simulink model "o03M_POROWNANIE_CIAGLY_DYSKRETNY_EULER"  (R2023a)
settings: Solver=ode45  StartTime=0.0  StopTime=5  RelTol=1e-3
values from neighbouring files (symbols this model uses):
  calka_on_off = 1    [o03S_skrypt_prownanie.m]
  den_f_e = sym2poly(d)    [o03S_skrypt_prownanie.m]
  fsz = 2500    [o03S_skrypt_prownanie.m]
  Jeq = JL + J    (= 3.228252e-05)    [o03S_skrypt_prownanie.m]
  K_windup = 3    [o03S_skrypt_prownanie.m]
  Km = 0.0257    [o03S_skrypt_prownanie.m]
  Kp = 0.04    [o03S_skrypt_prownanie.m]
  num_f_e = sym2poly(n)    [o03S_skrypt_prownanie.m]
  Psz = 0.005    [o03S_skrypt_prownanie.m]
  Rm = 2.675    [o03S_skrypt_prownanie.m]
  Td = 0.009    [o03S_skrypt_prownanie.m]
  Ti = 0.11    [o03S_skrypt_prownanie.m]
  Ts = 1/fs    (= 0.0333333333333)    [o03S_skrypt_prownanie.m]
  w_filtr = 10    [o03S_skrypt_prownanie.m]
undefined symbols (not defined in the file or in its folder): sigbuilder_block
libraries: simulink x2
settings Model: Creator=Adam  LastModifiedBy=Adam
settings SolverCC: ZeroCrossAlgorithm=Adaptive  AlgebraicLoopSolver=TrustRegion
settings DebuggingCC: IgnoredZcDiagnostic=none  UnconnectedInputMsg=warning  UnconnectedOutputMsg=warning  UnconnectedLineMsg=warning
settings ModelReferenceCC: EnableRefExpFcnMdlSchedulingChecks=on
settings RTWCC: DLArmComputeVersion=19.05

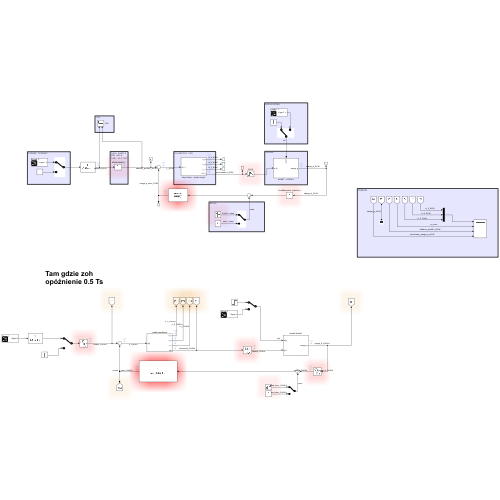
[thumbnail: Simulink's stored preview of the top-level diagram]
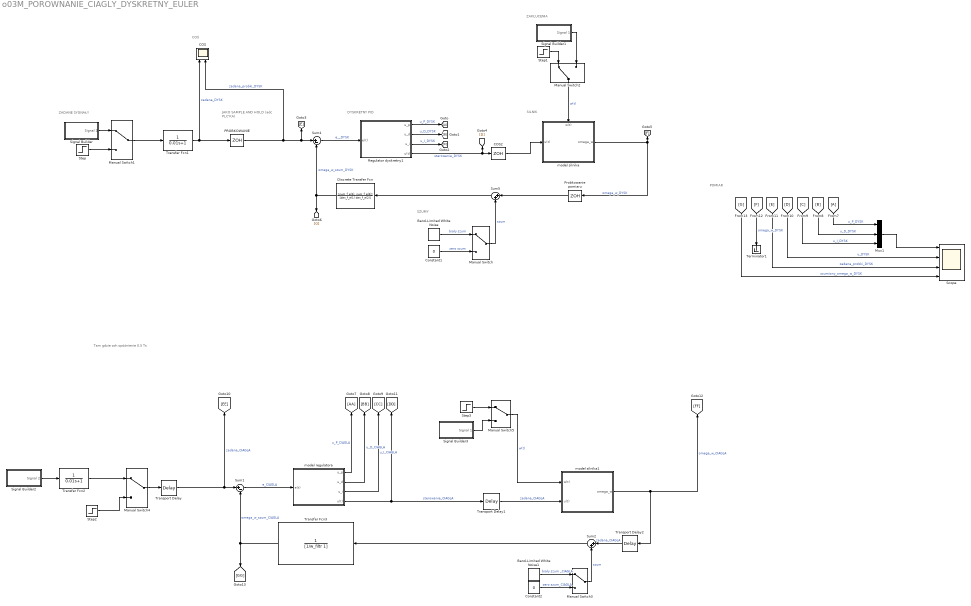
== system o03M_POROWNANIE_CIAGLY_DYSKRETNY_EULER ==
  note: Tam gdzie zoh opóźnienie 0.5 Ts
  note: ZAKŁUCENIA
  note: POMIAR
  note: SZUMY
  note: JAKO SAMPLE
      | AND HOLD
      | (adc PLC'KA)
  note: SILNIK
  note: DYSKRETNY PID
  note: COŚ
  note: ZADANE SYGNAŁY
  Band-Limited White Noise : simulink/Sources/Band-Limited White Noise  Cov=[Psz]  Ts=0.1  seed=[fsz]
  Band-Limited White Noise1 : simulink/Sources/Band-Limited White Noise  Cov=[Psz]  Ts=0.1  seed=[fsz]
  "COS " : Scope  NumInputPorts=2
  COS2 : ZeroOrderHold  SampleTime=Ts
  Constant1 : Constant  Value=0
  Constant2 : Constant  Value=0
  Discrete Transfer Fcn : DiscreteTransferFcn  Numerator=[num_f_e(1), num_f_e(2)]  Denominator=[den_f_e(1) den_f_e(2)]  SampleTime=Ts
  From7 : From
  Goto : Goto
  Manual Switch{,1..5} (6 alike) : ManualSwitch
  Mux1 : Mux  Inputs=3
  PROBKOWANIE : ZeroOrderHold  SampleTime=Ts
  Probkowanie pomiaru : ZeroOrderHold  SampleTime=Ts
  Regulator dyskretny1 : Subsystem
  Scope : Scope  NumInputPorts=4
  Signal Builder : Subsystem  Tag=STV Subsys  LoadFcn=sigbuilder_block('load');  StartFcn=sigbuilder_block('start');  StopFcn=sigbuilder_block('stop');  ClipboardFcn=sigbuilder_block('clipboard');  mask(Sigbuilder block){tuvar=[0:10]}
      mask help: Simulink:masks:SigbuilderBlock_MD
      mask init:
      | if ~strcmp(get_param(bdroot(gcbh),'SimulationStatus'),'stopped') tuvar = sigbuilder_block('maskInit'); end
      settings: CopyFcn=sigbuilder_block('copy');  DeleteFcn=sigbuilder_block('delete');  ModelCloseFcn=sigbuilder_block('modelClose');  PreSaveFcn=sigbuilder_block('preSave');  PauseFcn=sigbuilder_block('pause');  ContinueFcn=sigbuilder_block('continue');  NameChangeFcn=sigbuilder_block('namechange');  OpenFcn=sigbuilder_block('open',[261 231 1018.5 399.75 ]);  CloseFcn=sigbuilder_block('close');
      mask Display: plot(0, 0, 100, 100,[2, 2, 32, 32, 2], [68, 8, 8, 68, 68],[32, 2], [38, 38], [32, 19, 2],[53, 60, 44], [32, 17, 17, 2],[16, 16, 31, 31]);txt = getActiveGroup(gcbh);text(2, 100, txt,'verticalAlignment', 'top');
  Signal Builder1 : Subsystem  Tag=STV Subsys  LoadFcn=sigbuilder_block('load');  StartFcn=sigbuilder_block('start');  StopFcn=sigbuilder_block('stop');  ClipboardFcn=sigbuilder_block('clipboard');  mask(Sigbuilder block){tuvar=[0:10]}
      mask help: Simulink:masks:SigbuilderBlock_MD
      mask init:
      | if ~strcmp(get_param(bdroot(gcbh),'SimulationStatus'),'stopped') tuvar = sigbuilder_block('maskInit'); end
      settings: CopyFcn=sigbuilder_block('copy');  DeleteFcn=sigbuilder_block('delete');  ModelCloseFcn=sigbuilder_block('modelClose');  PreSaveFcn=sigbuilder_block('preSave');  PauseFcn=sigbuilder_block('pause');  ContinueFcn=sigbuilder_block('continue');  NameChangeFcn=sigbuilder_block('namechange');  OpenFcn=sigbuilder_block('open',[261 231 1018.5 399.75 ]);  CloseFcn=sigbuilder_block('close');
      mask Display: plot(0, 0, 100, 100,[2, 2, 32, 32, 2], [68, 8, 8, 68, 68],[32, 2], [38, 38], [32, 19, 2],[53, 60, 44], [32, 17, 17, 2],[16, 16, 31, 31]);txt = getActiveGroup(gcbh);text(2, 100, txt,'verticalAlignment', 'top');
  Signal Builder2 : Subsystem  Tag=STV Subsys  LoadFcn=sigbuilder_block('load');  StartFcn=sigbuilder_block('start');  StopFcn=sigbuilder_block('stop');  ClipboardFcn=sigbuilder_block('clipboard');  mask(Sigbuilder block){tuvar=[0:10]}
      mask help: Simulink:masks:SigbuilderBlock_MD
      mask init:
      | if ~strcmp(get_param(bdroot(gcbh),'SimulationStatus'),'stopped') tuvar = sigbuilder_block('maskInit'); end
      settings: CopyFcn=sigbuilder_block('copy');  DeleteFcn=sigbuilder_block('delete');  ModelCloseFcn=sigbuilder_block('modelClose');  PreSaveFcn=sigbuilder_block('preSave');  PauseFcn=sigbuilder_block('pause');  ContinueFcn=sigbuilder_block('continue');  NameChangeFcn=sigbuilder_block('namechange');  OpenFcn=sigbuilder_block('open',[261 231 1018.5 399.75 ]);  CloseFcn=sigbuilder_block('close');
      mask Display: plot(0, 0, 100, 100,[2, 2, 32, 32, 2], [68, 8, 8, 68, 68],[32, 2], [38, 38], [32, 19, 2],[53, 60, 44], [32, 17, 17, 2],[16, 16, 31, 31]);txt = getActiveGroup(gcbh);text(2, 100, txt,'verticalAlignment', 'top');
  Signal Builder3 : Subsystem  Tag=STV Subsys  LoadFcn=sigbuilder_block('load');  StartFcn=sigbuilder_block('start');  StopFcn=sigbuilder_block('stop');  ClipboardFcn=sigbuilder_block('clipboard');  mask(Sigbuilder block){tuvar=[0:10]}
      mask help: Simulink:masks:SigbuilderBlock_MD
      mask init:
      | if ~strcmp(get_param(bdroot(gcbh),'SimulationStatus'),'stopped') tuvar = sigbuilder_block('maskInit'); end
      settings: CopyFcn=sigbuilder_block('copy');  DeleteFcn=sigbuilder_block('delete');  ModelCloseFcn=sigbuilder_block('modelClose');  PreSaveFcn=sigbuilder_block('preSave');  PauseFcn=sigbuilder_block('pause');  ContinueFcn=sigbuilder_block('continue');  NameChangeFcn=sigbuilder_block('namechange');  OpenFcn=sigbuilder_block('open',[261 231 1018.5 399.75 ]);  CloseFcn=sigbuilder_block('close');
      mask Display: plot(0, 0, 100, 100,[2, 2, 32, 32, 2], [68, 8, 8, 68, 68],[32, 2], [38, 38], [32, 19, 2],[53, 60, 44], [32, 17, 17, 2],[16, 16, 31, 31]);txt = getActiveGroup(gcbh);text(2, 100, txt,'verticalAlignment', 'top');
  Step : Step  SampleTime=0
  Step1 : Step  Time=2  After=0.03  SampleTime=0
  Step2 : Step  SampleTime=0
  Step3 : Step  Time=2  After=0.03  SampleTime=0
  Sum1 : Sum  Inputs=|+-
  Sum2 : Sum  Inputs=|++
  Sum4 : Sum  Inputs=|+-
  Sum5 : Sum  Inputs=|++
  Terminator1 : Terminator
  Transfer Fcn1 : TransferFcn  Denominator=[0.01 1]
  Transfer Fcn2 : TransferFcn  Denominator=[0.01 1]
  Transfer Fcn3 : TransferFcn  Denominator=[1/w_filtr 1]
  Transport Delay : TransportDelay  DelayTime=Ts/2
  Transport Delay1 : TransportDelay  DelayTime=Ts/2
  Transport Delay2 : TransportDelay  DelayTime=Ts/2
  model regulatora : Subsystem
  model silnika : Subsystem
      settings: PortSchema="{\"entries\":[{\"content\":{\"sides\":[{\"content\":{\"connectorIds\":[\"In1\"]},\"type\":\"ConnectorPlacement.EquallySpacedRectSide\",\"uuid\":\"98491aef-0591-4405-8c9c-40e364f6fd31\"},{\"content\":{\"connectorIds\":[\"Out1\"],\"side\":\"RIGHT\"},\"type\":\"ConnectorPlacement.EquallySpacedRectSide\",\"uuid\":\"a1d3aa00-38e6-4d5e-ba9e-ca8054307f42\"},{\"content\":{\"connectorIds\":[\"In2\"],\"side\":\"TOP\"},\"type\":\"ConnectorPlacement.EquallySpacedRectSide\",\"uuid\":\"056a3762-abf1-4492-b9c7-e5ea07edcbab\"},{\"content\":{\"connectorIds\":[],\"side\":\"HIDDEN\"},\"type\":\"ConnectorPlacement.EquallySpacedRectSide\",\"uuid\":\"0c2ff021-be20-4132-8d80-585248c3a111\"}]},\"type\":\"ConnectorPlacement.EquallySpacedConnector\",\"uuid\":\"f7102573-6331-4f02-a900-8db50f80a4fd\"}],\"packageUris\":[\"http://schema.mathworks.com/mf0/Connector/R2020b\"],\"version\":\"1.0\"}"
  model silnika1 : Subsystem
  wires:
  Band-Limited White Noise/1 -> Manual Switch/1  "biały szum"
  Constant1/1 -> Manual Switch/2  "zero szum"
  model silnika/1(omega_w) -> Probkowanie pomiaru/1, [F]  "omega_w_DYSK"
  Manual Switch/1 -> Sum5/2  "szum"
  Signal Builder/1(Signal 2) -> Manual Switch1/1
  Step/1 -> Manual Switch1/2
  [G] -> Scope/4  "szumiony_omega_w_DYSK"
  [C] -> Mux1/3  "u_I_DYSK"
  [E] -> Scope/3  "zadana_probki_DYSK"
  [D] -> Scope/2  "u_DYSK"
  From7/1 -> Mux1/1  "u_P_DYSK"
  [B] -> Mux1/2  "u_D_DYSK"
  Mux1/1 -> Scope/1
  [F] -> Terminator1/1  "omega_w_DYSK"
  Regulator dyskretny1/3(u_i) -> [C]  "u_I_DYSK"
  Regulator dyskretny1/1(u_p) -> Goto/1  "u_P_DYSK"
  Regulator dyskretny1/4(u(t)) -> [D], COS2/1  "sterowanie_DYSK"
  Sum4/1 -> Regulator dyskretny1/1(e(t))  "e__DYSK"
  Regulator dyskretny1/2(u_d) -> [B]  "u_D_DYSK"
  Sum5/1 -> Discrete Transfer Fcn/1
  Step1/1 -> Manual Switch2/1
  Signal Builder1/1(Signal 1) -> Manual Switch2/2
  PROBKOWANIE/1 -> "COS "/2, Sum4/1, [E]  "zadana_probki_DYSK"
  Probkowanie pomiaru/1 -> Sum5/1
  COS2/1 -> model silnika/1(u(t))
  Transfer Fcn1/1 -> PROBKOWANIE/1, "COS "/1  "zadana_DYSK"
  Manual Switch1/1 -> Transfer Fcn1/1
  Manual Switch2/1 -> model silnika/2(w(t))  "w(t)"
  Discrete Transfer Fcn/1 -> [G], Sum4/2  "omega_w_szum_DYSK"
  Sum1/1 -> model regulatora/1(e(t))  "e_CIAGLA"
  model silnika1/1(omega_w) -> Transport Delay2/1, [FF]  "omega_w_CIAGLA"
  Manual Switch5/1 -> model silnika1/1(w(t))  "w(t)"
  Constant2/1 -> Manual Switch3/2  "zero szum_CIAGLA"
  Signal Builder3/1(Signal 1) -> Manual Switch5/2
  model regulatora/1(u_p) -> [AA]  "u_P_CIAGLA"
  Step2/1 -> Manual Switch4/2
  Signal Builder2/1(Signal 2) -> Transfer Fcn2/1
  Manual Switch3/1 -> Sum2/2  "szum"
  Transfer Fcn2/1 -> Manual Switch4/1
  model regulatora/2(u_d) -> [BB]  "u_D_CIAGLA"
  Step3/1 -> Manual Switch5/1
  Transfer Fcn3/1 -> [GG], Sum1/2  "omega_w_szum_CIAGLA"
  model regulatora/3(u_i) -> [CC]  "u_I_CIAGLA"
  model regulatora/4(u(t)) -> [DD], Transport Delay1/1  "sterowanie_CIAGLA"
  Manual Switch4/1 -> Transport Delay/1
  Sum2/1 -> Transfer Fcn3/1
  Band-Limited White Noise1/1 -> Manual Switch3/1  "biały szum _CIAGLA"
  Transport Delay/1 -> [EE], Sum1/1  "zadana_CIAGLA"
  Transport Delay1/1 -> model silnika1/2(u(t))  "zadana_CIAGLA"
  Transport Delay2/1 -> Sum2/1  "zadana_CIAGLA"

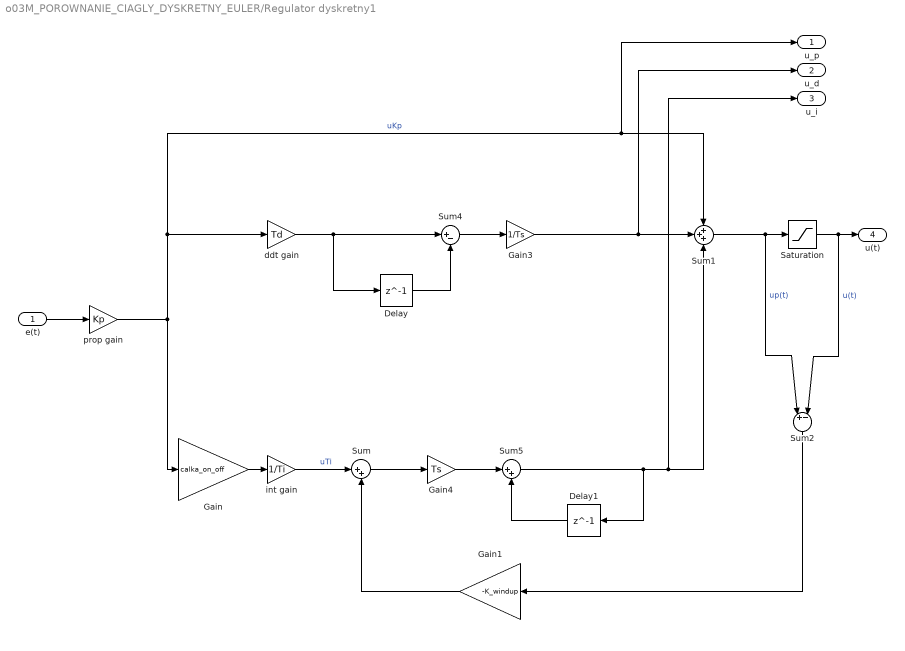
== system o03M_POROWNANIE_CIAGLY_DYSKRETNY_EULER/Regulator dyskretny1 ==
  e(t) : Inport
  Delay : Delay  DelayLength=1  SampleTime=Ts
  Delay1 : Delay  DelayLength=1  SampleTime=Ts
  Gain : Gain  Gain=calka_on_off
  Gain1 : Gain  Gain=-K_windup
  Gain3 : Gain  Gain=1/Ts
  Gain4 : Gain  Gain=Ts
  Saturation : Saturate  UpperLimit=10  LowerLimit=-10  ZeroCross=off
  Sum : Sum  Inputs=|++
  Sum1 : Sum  Inputs=+++
  Sum2 : Sum  Inputs=|+-|
  Sum4 : Sum  Inputs=|+-
  Sum5 : Sum  Inputs=|++
  ddt gain : Gain  Gain=Td
  int gain : Gain  Gain=1/Ti
  prop gain : Gain  Gain=Kp
  u_p : Outport
  u_d : Outport  Port=2
  u_i : Outport  Port=3
  u(t) : Outport  Port=4
  wires:
  Sum1/1 -> Sum2/1, Saturation/1  "up(t)"
  prop gain/1 -> Sum1/1, u_p/1, ddt gain/1, Gain/1  "uKp"
  Saturation/1 -> Sum2/2, u(t)/1  "u(t)"
  e(t)/1 -> prop gain/1
  Gain/1 -> int gain/1
  int gain/1 -> Sum/1  "uTi"
  Gain1/1 -> Sum/2
  Sum2/1 -> Gain1/1
  ddt gain/1 -> Delay/1, Sum4/1
  Delay/1 -> Sum4/2
  Sum4/1 -> Gain3/1
  Sum/1 -> Gain4/1
  Gain3/1 -> u_d/1, Sum1/2
  Gain4/1 -> Sum5/1
  Delay1/1 -> Sum5/2
  Sum5/1 -> Delay1/1, u_i/1, Sum1/3

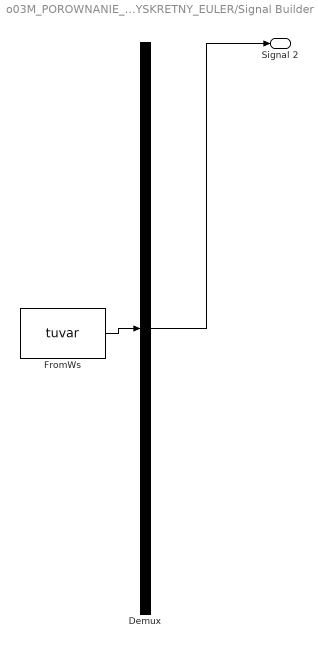
== system o03M_POROWNANIE_CIAGLY_DYSKRETNY_EULER/Signal Builder ==
  Demux : Demux  Tag=STV Demux  Outputs=1
      settings: DisplayOption=none
  FromWs : FromWorkspace  Tag=STV FromWs  VariableName=tuvar
      SigBuilderData=|
      | common.afterFinalStr = 'Extrapolate'
      | common.sampleTime = 0
      | dataSet.timeRange = [0 25]
      | dataSet.name = 'Group 1'
      | sbobj.Groups.Name = 'Group 1'
      | sbobj.Groups.Signals.Name = 'Signal 2'
      | sbobj.Groups.Signals.XData = [0 4 4 9.2 9.2 14 14 25]
      | sbobj.Groups.Signals.YData = [100 100 -150 -150 -100 -100 150 150]
      | sbobj.Groups.TimeRange = [0 25]
  Signal 2 : Outport  Tag=STV Outport
  wires:
  FromWs/1 -> Demux/1
  Demux/1 -> Signal 2/1

== system o03M_POROWNANIE_CIAGLY_DYSKRETNY_EULER/Signal Builder1 ==
  Demux : Demux  Tag=STV Demux  Outputs=1
      settings: DisplayOption=none
  FromWs : FromWorkspace  Tag=STV FromWs  VariableName=tuvar
      SigBuilderData=|
      | common.afterFinalStr = 'Extrapolate'
      | common.sampleTime = 0
      | dataSet.timeRange = [0 25]
      | dataSet.name = 'Group 1'
      | sbobj.Groups.Name = 'Group 1'
      | sbobj.Groups.Signals.Name = 'Signal 1'
      | sbobj.Groups.Signals.XData = [0 2.05 2.05 4.05 4.05 6 6 8 8 16 16 18 18 25]
      | sbobj.Groups.Signals.YData = [0 0 0.075 0.075 -0.001 -0.001 -0.0775 -0.0775 0 0 0.075 0.075 0 0]
      | sbobj.Groups.TimeRange = [0 25]
  Signal 1 : Outport  Tag=STV Outport
  wires:
  FromWs/1 -> Demux/1
  Demux/1 -> Signal 1/1

== system o03M_POROWNANIE_CIAGLY_DYSKRETNY_EULER/Signal Builder2 ==
  Demux : Demux  Tag=STV Demux  Outputs=1
      settings: DisplayOption=none
  FromWs : FromWorkspace  Tag=STV FromWs  VariableName=tuvar
      SigBuilderData=|
      | common.afterFinalStr = 'Extrapolate'
      | common.sampleTime = 0
      | dataSet.timeRange = [0 25]
      | dataSet.name = 'Group 1'
      | sbobj.Groups.Name = 'Group 1'
      | sbobj.Groups.Signals.Name = 'Signal 2'
      | sbobj.Groups.Signals.XData = [0 4 4 9.2 9.2 14 14 25]
      | sbobj.Groups.Signals.YData = [100 100 -150 -150 -100 -100 150 150]
      | sbobj.Groups.TimeRange = [0 25]
  Signal 2 : Outport  Tag=STV Outport
  wires:
  FromWs/1 -> Demux/1
  Demux/1 -> Signal 2/1

== system o03M_POROWNANIE_CIAGLY_DYSKRETNY_EULER/Signal Builder3 ==
  Demux : Demux  Tag=STV Demux  Outputs=1
      settings: DisplayOption=none
  FromWs : FromWorkspace  Tag=STV FromWs  VariableName=tuvar
      SigBuilderData=|
      | common.afterFinalStr = 'Extrapolate'
      | common.sampleTime = 0
      | dataSet.timeRange = [0 25]
      | dataSet.name = 'Group 1'
      | sbobj.Groups.Name = 'Group 1'
      | sbobj.Groups.Signals.Name = 'Signal 1'
      | sbobj.Groups.Signals.XData = [0 2.05 2.05 4.05 4.05 6 6 8 8 16 16 18 18 25]
      | sbobj.Groups.Signals.YData = [0 0 0.075 0.075 -0.001 -0.001 -0.0775 -0.0775 0 0 0.075 0.075 0 0]
      | sbobj.Groups.TimeRange = [0 25]
  Signal 1 : Outport  Tag=STV Outport
  wires:
  FromWs/1 -> Demux/1
  Demux/1 -> Signal 1/1

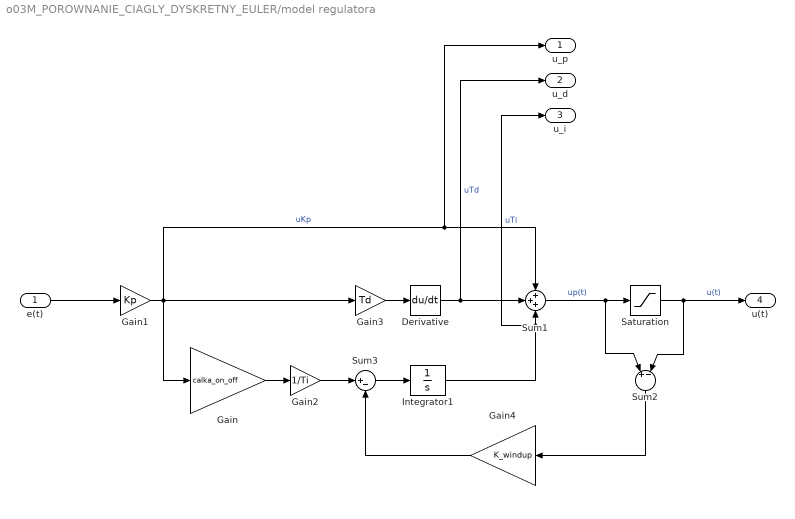
== system o03M_POROWNANIE_CIAGLY_DYSKRETNY_EULER/model regulatora ==
  e(t) : Inport
  Derivative : Derivative  CoefficientInTFapproximation=500
  Gain : Gain  Gain=calka_on_off
  Gain1 : Gain  Gain=Kp
  Gain2 : Gain  Gain=1/Ti
  Gain3 : Gain  Gain=Td
  Gain4 : Gain  Gain=K_windup
  Integrator1 : Integrator
  Saturation : Saturate  UpperLimit=10  LowerLimit=-10  ZeroCross=off
  Sum1 : Sum  Inputs=+++
  Sum2 : Sum  Inputs=|+-|
  Sum3 : Sum  Inputs=|+-
  u_p : Outport
  u_d : Outport  Port=2
  u_i : Outport  Port=3
  u(t) : Outport  Port=4
  wires:
  Sum1/1 -> Sum2/1, Saturation/1  "up(t)"
  Gain2/1 -> Sum3/1
  Sum2/1 -> Gain4/1
  Derivative/1 -> u_d/1, Sum1/2  "uTd"
  Gain3/1 -> Derivative/1
  Gain1/1 -> Gain/1, Gain3/1, u_p/1, Sum1/1  "uKp"
  Integrator1/1 -> u_i/1, Sum1/3  "uTi"
  Sum3/1 -> Integrator1/1
  Saturation/1 -> u(t)/1, Sum2/2  "u(t)"
  e(t)/1 -> Gain1/1
  Gain/1 -> Gain2/1
  Gain4/1 -> Sum3/2

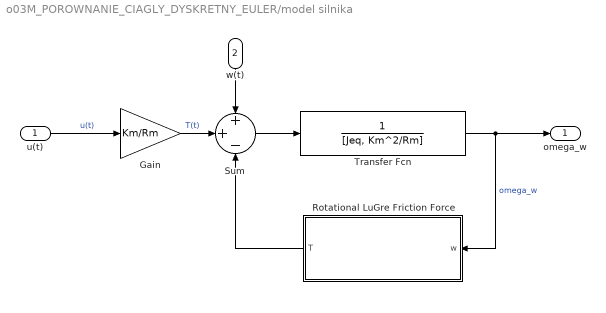
== system o03M_POROWNANIE_CIAGLY_DYSKRETNY_EULER/model silnika ==
  u(t) : Inport
  w(t) : Inport  Port=2
  Gain : Gain  Gain=Km/Rm
  Rotational LuGre Friction Force : Subsystem  TreatAsAtomicUnit=on  mask(LuGre friction model){ro0=1.2, ro1=0.05, ro2=2.9e-6, Fc=0.77e-3, Fs=12e-3, Vs=0.09}
      mask prompts: Fc "Culomb force (Fc)"; Fs "Friction force (Fs)"; Vs "Striback velocity (Vs)"
      mask help:
      | The LuGre model is a dynamic friction model. The model is related to the bristle interpretation of friction. Friction is modeled as the average deflection force of elastic springs. When a tangential force is applied the bristles will deflect like springs. If the deflection is sufficiently large the bristles start to slip.
      |
      | The input signal is the velocity of the object. The output signal is the fristion force value.
      mask Help:
      | <!DOCTYPE html   PUBLIC "-//W3C//DTD HTML 4.01 Transitional//EN" "http://www.w3.org/TR/1999/REC-html401-19991224/loose.dtd">
      | <html lang="en"><head>
      | <meta http-equiv="Content-Type" content="text/html; charset=utf-8">
      | <title>About :: LuGre friction model</title>
      | <meta name="description" content="">
      | </head>
      | <body><a name="top_of_page"></a>
      | The LuGre model is a dynamic friction model. The model is related to
      | the bristle interpretation of friction. Friction is modeled as the average
      | deflection force of elastic springs. When a tangential force is applied the bristles
      | will deflect like springs. If the deflection is sufficiently large the bristles start
      | to slip. The average bristle deflection for a steady state motion is determined
      | by the velocity. It is lower at low velocities, which implies that the steady state
      | deflection decreases with increasing velocity. This models the phenomenon that
      | the surfaces are pushed apart by the lubricant, and models the Stribeck effect.
      | The model also includes rate dependent friction phenomena such as varying
      | break-away force and frictional lag.<sup><a href="#ref1">1</a></sup></p><p>More information about the model may be found in the labsheets.</p>
      | <hr><small>
      | <sup><a name="ref1"></a>1</sup> <b>Friction Models and Friction Compensation</b>. H. Olsson, K.J. &Aring;str&ouml;m, C. Canudas de Wit, M. G&auml;fvert, P. Lischinsky
      | </small>
      | <br />
      | <br />
      | <hr>
      | <center><small>Copyright&copy;2009
      | <a href="mailto:w.kurek@ely.pg.gda.pl">Wojciech Kurek</a>,
      | <a href="mailto:g.ewald@ely.pg.gda.pl">Grzegorz Ewald</a>
      | </small></center>
      | </body>
      | </html>
      mask Callback ro0:
      | if str2num(get_param(gcb, 'ro0')) <= 0
      |     error('ro0 is negative!')
      | end
      mask Callback ro1:
      | if str2num(get_param(gcb, 'ro1')) <= 0
      |     error('ro1 is negative!')
      | end
      mask Callback ro2:
      | if str2num(get_param(gcb, 'ro2')) <= 0
      |     error('ro2 is negative!')
      | end
      mask Callback Fc:
      | if str2num(get_param(gcb, 'Fs')) <= 0
      |     error('Culomb force is negative!')
      | end
      mask Callback Fs:
      | if str2num(get_param(gcb, 'Fs')) <= 0
      |     error('Friction force is negative!')
      | end
      mask Callback Vs:
      | if str2num(get_param(gcb, 'Vs')) <= 0
      |     error('Striback velocity is negative!')
      | end
      mask Display:
      | patch([0.1 0.1 0.9 0.9],[0.1 0.25 0.25 0.1],[0.8 0.8 0.8])
      | patch([0.1 0.1 0.9 0.9],[0.9 0.75 0.75 0.9],[0.8 0.8 0.8])
      | 
      | plot([0.12 0.12],[0.25 0.5])
      | plot([0.2 0.2],[0.25 0.5])
      | plot([0.4 0.4],[0.25 0.5])
      | plot([0.57 0.57],[0.25 0.5])
      | plot([0.67 0.67],[0.25 0.5])
      | plot([0.87 0.87],[0.25 0.5])
      | 
      | plot([0.17 0.18 0.2 0.23],[0.75 0.6 0.5 0.45])
      | plot([0.35 0.36 0.39 0.44],[0.75 0.6 0.5 0.48])
      | plot([0.62 0.64 0.68 0.72],[0.75 0.6 0.5 0.48])
      | plot([0.85 0.86 0.87 0.89],[0.75 0.6 0.5 0.48])
      | 
      | plot([0.15 0.15],[0.75 0.4])
      | plot([0.28 0.28],[0.75 0.4])
      | plot([0.55 0.55],[0.75 0.4])
      | plot([0.8 0.8],[0.75 0.4])
      | 
      | color('blue');
      | port_label('input',1,'\omega','texmode','on')
      | port_label('output',1,'T','texmode','on')
  Sum : Sum  Inputs=++-
  Transfer Fcn : TransferFcn  Denominator=[Jeq, Km^2/Rm]
  omega_w : Outport
  wires:
  Transfer Fcn/1 -> Rotational LuGre Friction Force/1(w), omega_w/1  "omega_w"
  Rotational LuGre Friction Force/1(T) -> Sum/3
  Sum/1 -> Transfer Fcn/1
  Gain/1 -> Sum/2  "T(t)"
  u(t)/1 -> Gain/1  "u(t)"
  w(t)/1 -> Sum/1

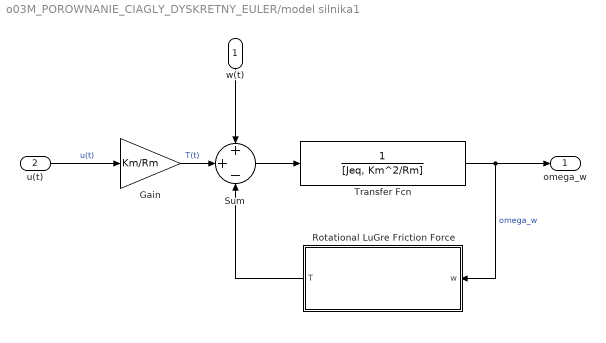
== system o03M_POROWNANIE_CIAGLY_DYSKRETNY_EULER/model silnika1 ==
  w(t) : Inport
  u(t) : Inport  Port=2
  Gain : Gain  Gain=Km/Rm
  Rotational LuGre Friction Force : Subsystem  TreatAsAtomicUnit=on  mask(LuGre friction model){ro0=1.2, ro1=0.05, ro2=2.9e-6, Fc=0.77e-3, Fs=12e-3, Vs=0.09}
      mask prompts: Fc "Culomb force (Fc)"; Fs "Friction force (Fs)"; Vs "Striback velocity (Vs)"
      mask help:
      | The LuGre model is a dynamic friction model. The model is related to the bristle interpretation of friction. Friction is modeled as the average deflection force of elastic springs. When a tangential force is applied the bristles will deflect like springs. If the deflection is sufficiently large the bristles start to slip.
      |
      | The input signal is the velocity of the object. The output signal is the fristion force value.
      mask Help:
      | <!DOCTYPE html   PUBLIC "-//W3C//DTD HTML 4.01 Transitional//EN" "http://www.w3.org/TR/1999/REC-html401-19991224/loose.dtd">
      | <html lang="en"><head>
      | <meta http-equiv="Content-Type" content="text/html; charset=utf-8">
      | <title>About :: LuGre friction model</title>
      | <meta name="description" content="">
      | </head>
      | <body><a name="top_of_page"></a>
      | The LuGre model is a dynamic friction model. The model is related to
      | the bristle interpretation of friction. Friction is modeled as the average
      | deflection force of elastic springs. When a tangential force is applied the bristles
      | will deflect like springs. If the deflection is sufficiently large the bristles start
      | to slip. The average bristle deflection for a steady state motion is determined
      | by the velocity. It is lower at low velocities, which implies that the steady state
      | deflection decreases with increasing velocity. This models the phenomenon that
      | the surfaces are pushed apart by the lubricant, and models the Stribeck effect.
      | The model also includes rate dependent friction phenomena such as varying
      | break-away force and frictional lag.<sup><a href="#ref1">1</a></sup></p><p>More information about the model may be found in the labsheets.</p>
      | <hr><small>
      | <sup><a name="ref1"></a>1</sup> <b>Friction Models and Friction Compensation</b>. H. Olsson, K.J. &Aring;str&ouml;m, C. Canudas de Wit, M. G&auml;fvert, P. Lischinsky
      | </small>
      | <br />
      | <br />
      | <hr>
      | <center><small>Copyright&copy;2009
      | <a href="mailto:w.kurek@ely.pg.gda.pl">Wojciech Kurek</a>,
      | <a href="mailto:g.ewald@ely.pg.gda.pl">Grzegorz Ewald</a>
      | </small></center>
      | </body>
      | </html>
      mask Callback ro0:
      | if str2num(get_param(gcb, 'ro0')) <= 0
      |     error('ro0 is negative!')
      | end
      mask Callback ro1:
      | if str2num(get_param(gcb, 'ro1')) <= 0
      |     error('ro1 is negative!')
      | end
      mask Callback ro2:
      | if str2num(get_param(gcb, 'ro2')) <= 0
      |     error('ro2 is negative!')
      | end
      mask Callback Fc:
      | if str2num(get_param(gcb, 'Fs')) <= 0
      |     error('Culomb force is negative!')
      | end
      mask Callback Fs:
      | if str2num(get_param(gcb, 'Fs')) <= 0
      |     error('Friction force is negative!')
      | end
      mask Callback Vs:
      | if str2num(get_param(gcb, 'Vs')) <= 0
      |     error('Striback velocity is negative!')
      | end
      mask Display:
      | patch([0.1 0.1 0.9 0.9],[0.1 0.25 0.25 0.1],[0.8 0.8 0.8])
      | patch([0.1 0.1 0.9 0.9],[0.9 0.75 0.75 0.9],[0.8 0.8 0.8])
      | 
      | plot([0.12 0.12],[0.25 0.5])
      | plot([0.2 0.2],[0.25 0.5])
      | plot([0.4 0.4],[0.25 0.5])
      | plot([0.57 0.57],[0.25 0.5])
      | plot([0.67 0.67],[0.25 0.5])
      | plot([0.87 0.87],[0.25 0.5])
      | 
      | plot([0.17 0.18 0.2 0.23],[0.75 0.6 0.5 0.45])
      | plot([0.35 0.36 0.39 0.44],[0.75 0.6 0.5 0.48])
      | plot([0.62 0.64 0.68 0.72],[0.75 0.6 0.5 0.48])
      | plot([0.85 0.86 0.87 0.89],[0.75 0.6 0.5 0.48])
      | 
      | plot([0.15 0.15],[0.75 0.4])
      | plot([0.28 0.28],[0.75 0.4])
      | plot([0.55 0.55],[0.75 0.4])
      | plot([0.8 0.8],[0.75 0.4])
      | 
      | color('blue');
      | port_label('input',1,'\omega','texmode','on')
      | port_label('output',1,'T','texmode','on')
  Sum : Sum  Inputs=++-
  Transfer Fcn : TransferFcn  Denominator=[Jeq, Km^2/Rm]
  omega_w : Outport
  wires:
  Transfer Fcn/1 -> Rotational LuGre Friction Force/1(w), omega_w/1  "omega_w"
  Rotational LuGre Friction Force/1(T) -> Sum/3
  w(t)/1 -> Sum/1
  Sum/1 -> Transfer Fcn/1
  Gain/1 -> Sum/2  "T(t)"
  u(t)/1 -> Gain/1  "u(t)"

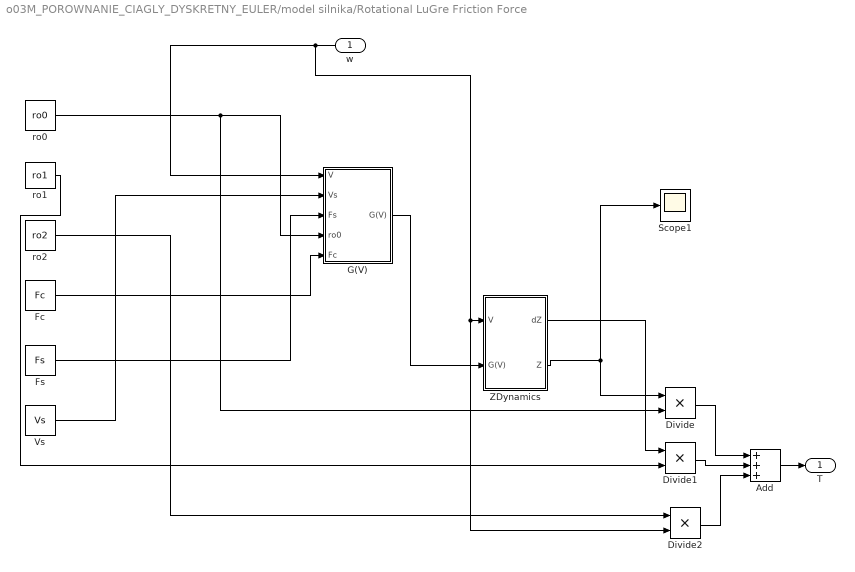
== system o03M_POROWNANIE_CIAGLY_DYSKRETNY_EULER/model silnika/Rotational LuGre Friction Force ==
  w : Inport
  Add : Sum  Inputs=+++
  Divide : Product  Inputs=**
  Divide1 : Product  Inputs=**
  Divide2 : Product  Inputs=**
  Fc : Constant  Value=Fc
  Fs : Constant  Value=Fs
  G(V) : Subsystem
  Scope1 : Scope
  Vs : Constant  Value=Vs
  ZDynamics : Subsystem
  ro0 : Constant  Value=ro0
  ro1 : Constant  Value=ro1
  ro2 : Constant  Value=ro2
  T : Outport
  wires:
  Add/1 -> T/1
  Divide2/1 -> Add/3
  Divide1/1 -> Add/2
  Divide/1 -> Add/1
  ro2/1 -> Divide2/1
  ro1/1 -> Divide1/2
  ZDynamics/1(dZ) -> Divide1/1
  ZDynamics/2(Z) -> Scope1/1, Divide/1
  G(V)/1(G(V)) -> ZDynamics/2(G(V))
  ro0/1 -> Divide/2, G(V)/4(ro0)
  Fc/1 -> G(V)/5(Fc)
  Fs/1 -> G(V)/3(Fs)
  Vs/1 -> G(V)/2(Vs)
  w/1 -> G(V)/1(V), ZDynamics/1(V), Divide2/2

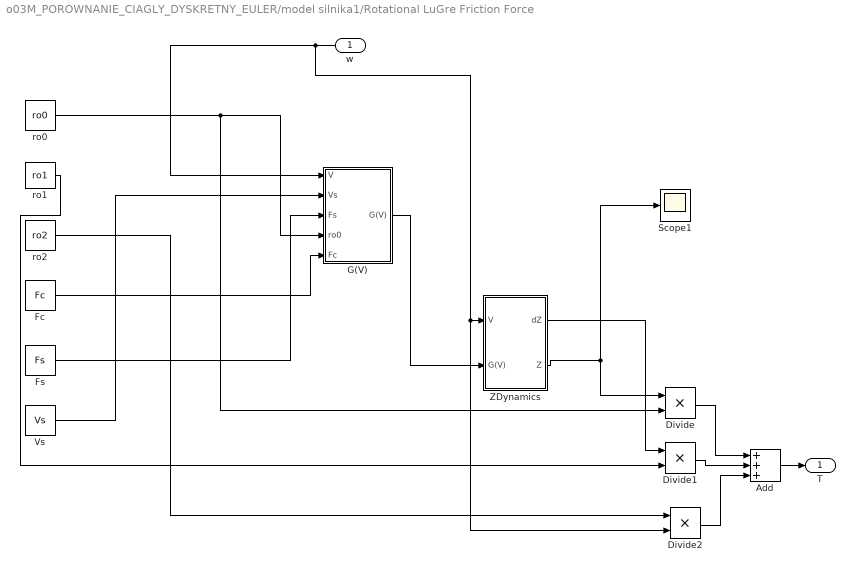
== system o03M_POROWNANIE_CIAGLY_DYSKRETNY_EULER/model silnika1/Rotational LuGre Friction Force ==
  w : Inport
  Add : Sum  Inputs=+++
  Divide : Product  Inputs=**
  Divide1 : Product  Inputs=**
  Divide2 : Product  Inputs=**
  Fc : Constant  Value=Fc
  Fs : Constant  Value=Fs
  G(V) : Subsystem
  Scope1 : Scope
  Vs : Constant  Value=Vs
  ZDynamics : Subsystem
  ro0 : Constant  Value=ro0
  ro1 : Constant  Value=ro1
  ro2 : Constant  Value=ro2
  T : Outport
  wires:
  Add/1 -> T/1
  Divide2/1 -> Add/3
  Divide1/1 -> Add/2
  Divide/1 -> Add/1
  ro2/1 -> Divide2/1
  ro1/1 -> Divide1/2
  ZDynamics/1(dZ) -> Divide1/1
  ZDynamics/2(Z) -> Scope1/1, Divide/1
  G(V)/1(G(V)) -> ZDynamics/2(G(V))
  ro0/1 -> Divide/2, G(V)/4(ro0)
  Fc/1 -> G(V)/5(Fc)
  Fs/1 -> G(V)/3(Fs)
  Vs/1 -> G(V)/2(Vs)
  w/1 -> G(V)/1(V), ZDynamics/1(V), Divide2/2

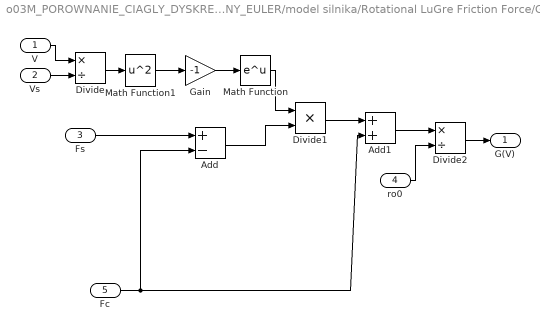
== system o03M_POROWNANIE_CIAGLY_DYSKRETNY_EULER/model silnika/Rotational LuGre Friction Force/G(V) ==
  V : Inport
  Vs : Inport  Port=2
  Fs : Inport  Port=3
  ro0 : Inport  Port=4
  Fc : Inport  Port=5
  Add : Sum  Inputs=+-
  Add1 : Sum
  Divide : Product  Inputs=*/
  Divide1 : Product  Inputs=**
  Divide2 : Product  Inputs=*/
  Gain : Gain  Gain=-1
  Math Function : Math  SignedPower=on
  Math Function1 : Math  Operator=square  SignedPower=on
  G(V) : Outport
  wires:
  Math Function/1 -> Divide1/1
  Gain/1 -> Math Function/1
  Math Function1/1 -> Gain/1
  ro0/1 -> Divide2/2
  Divide2/1 -> G(V)/1
  Fs/1 -> Add/1
  Vs/1 -> Divide/2
  V/1 -> Divide/1
  Add1/1 -> Divide2/1
  Divide1/1 -> Add1/1
  Add/1 -> Divide1/2
  Fc/1 -> Add/2, Add1/2
  Divide/1 -> Math Function1/1

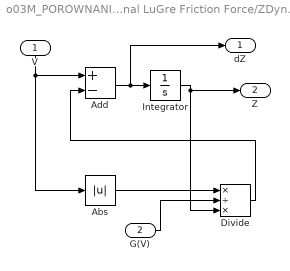
== system o03M_POROWNANIE_CIAGLY_DYSKRETNY_EULER/model silnika/Rotational LuGre Friction Force/ZDynamics ==
  V : Inport
  G(V) : Inport  Port=2
  Abs : Abs  SaturateOnIntegerOverflow=off
  Add : Sum  Inputs=+-
  Divide : Product  Inputs=*/*
  Integrator : Integrator
  dZ : Outport
  Z : Outport  Port=2
  wires:
  G(V)/1 -> Divide/2
  V/1 -> Abs/1, Add/1
  Divide/1 -> Add/2
  Integrator/1 -> Z/1, Divide/3
  Abs/1 -> Divide/1
  Add/1 -> dZ/1, Integrator/1

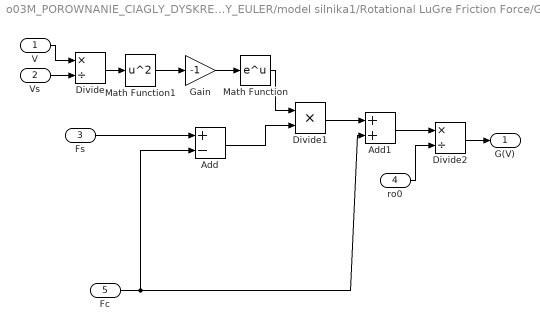
== system o03M_POROWNANIE_CIAGLY_DYSKRETNY_EULER/model silnika1/Rotational LuGre Friction Force/G(V) ==
  V : Inport
  Vs : Inport  Port=2
  Fs : Inport  Port=3
  ro0 : Inport  Port=4
  Fc : Inport  Port=5
  Add : Sum  Inputs=+-
  Add1 : Sum
  Divide : Product  Inputs=*/
  Divide1 : Product  Inputs=**
  Divide2 : Product  Inputs=*/
  Gain : Gain  Gain=-1
  Math Function : Math  SignedPower=on
  Math Function1 : Math  Operator=square  SignedPower=on
  G(V) : Outport
  wires:
  Math Function/1 -> Divide1/1
  Gain/1 -> Math Function/1
  Math Function1/1 -> Gain/1
  ro0/1 -> Divide2/2
  Divide2/1 -> G(V)/1
  Fs/1 -> Add/1
  Vs/1 -> Divide/2
  V/1 -> Divide/1
  Add1/1 -> Divide2/1
  Divide1/1 -> Add1/1
  Add/1 -> Divide1/2
  Fc/1 -> Add/2, Add1/2
  Divide/1 -> Math Function1/1

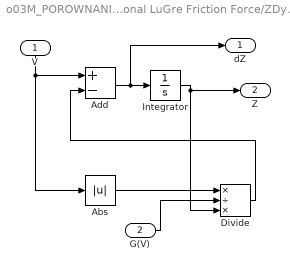
== system o03M_POROWNANIE_CIAGLY_DYSKRETNY_EULER/model silnika1/Rotational LuGre Friction Force/ZDynamics ==
  V : Inport
  G(V) : Inport  Port=2
  Abs : Abs  SaturateOnIntegerOverflow=off
  Add : Sum  Inputs=+-
  Divide : Product  Inputs=*/*
  Integrator : Integrator
  dZ : Outport
  Z : Outport  Port=2
  wires:
  G(V)/1 -> Divide/2
  V/1 -> Abs/1, Add/1
  Divide/1 -> Add/2
  Integrator/1 -> Z/1, Divide/3
  Abs/1 -> Divide/1
  Add/1 -> dZ/1, Integrator/1
